simulink model "DC_motor_Real_sys_open"  (R2021b)
settings: Solver=FixedStepAuto  StartTime=0.0  StopTime=10.0  RelTol=1e-3
undefined symbols (not defined in the file): sigbuilder_block
libraries: arduinolib x2, arduinosensorlib x1
settings Model: ExtModeTrigDuration=2  Creator=Marco Milanesi  LastModifiedBy=Marco Milanesi
settings OptimizationCC: EnhancedBackFolding=on  PassReuseOutputArgsAs=Individual arguments  ZeroExternalMemoryAtStartup=off  ZeroInternalMemoryAtStartup=off  MaxStackSize=64  OptimizeBlockOrder=speed  DifferentSizesBufferReuse=on  OptimizationCustomize=off  EfficientTunableParamExpr=on
settings DebuggingCC: ParameterTunabilityLossMsg=error
settings HardwareCC: ProdBitPerInt=16  ProdBitPerPointer=16  ProdBitPerSizeT=16  ProdBitPerPtrDiffT=16  ProdLargestAtomicFloat=None  ProdWordSize=8  ProdHWDeviceType=Atmel->AVR  UseEmbeddedCoderFeatures=off  UseSimulinkCoderFeatures=off
settings SFSimCC: MATLABDynamicMemAlloc=off
settings RTWCC: Description=Embedded Coder  SystemTargetFile=ert.tlc  HardwareBoard=Arduino Uno  TemplateMakefile=ert_default_tmf  Toolchain=Arduino AVR
settings CodeAppCC: ForceParamTrailComments=on  IgnoreCustomStorageClasses=off  OperatorAnnotations=on  SimulinkDataObjDesc=on  SFDataObjDesc=on  InsertBlockDesc=on
settings ERTTargetCC: SupportContinuousTime=on  SupportNonInlinedSFcns=on  SupportVariableSizeSignals=on  ExtModeTransport=3  ExtModeStaticAlloc=on  ExtModeStaticAllocSize=250  ExtModeMexFile=ext_xcp  ExtModeIntrfLevel=Level2 - Open

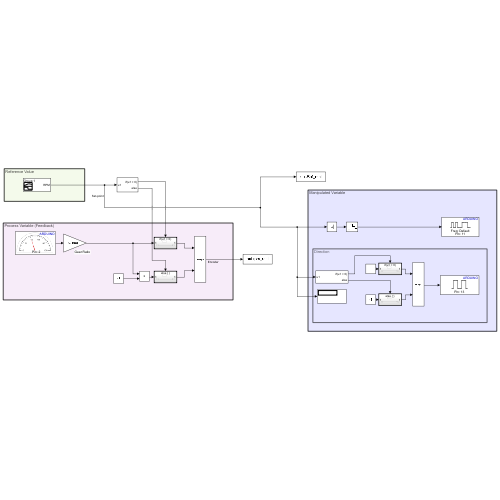
[thumbnail: Simulink's stored preview of the top-level diagram]
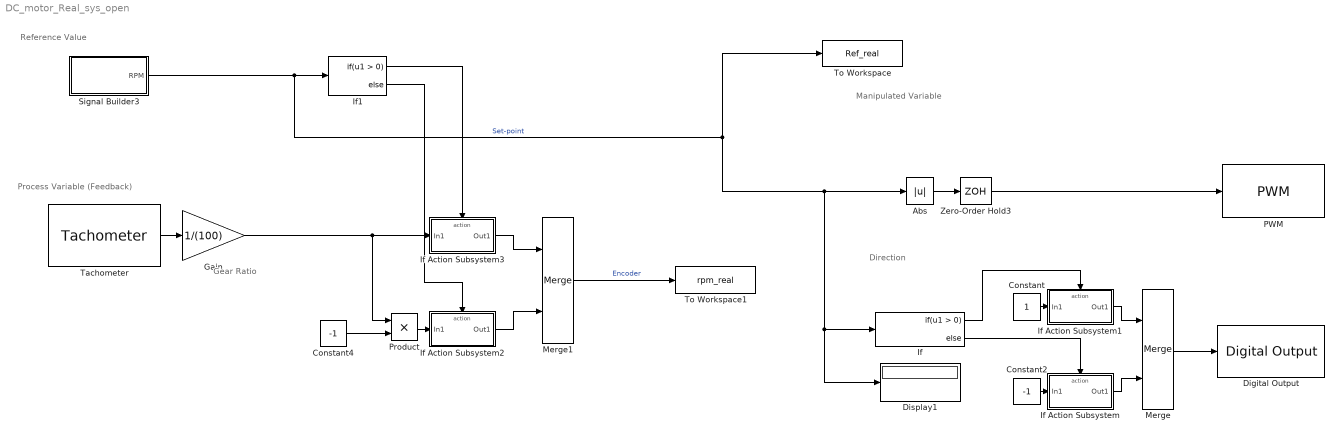
== system DC_motor_Real_sys_open ==
  note: Reference Value
  note: Process Variable (Feedback)
  note: Direction
  note: Manipulated Variable
  note: Gear Ratio
  Abs : Abs
  Constant : Constant
  Constant2 : Constant  Value=-1
  Constant4 : Constant  Value=-1
  Digital Output : arduinolib/Digital Output  pinNumber=13  Direction=output  blockPlatform=arduino
  Display1 : Display
  Gain : Gain  Gain=1/(100)  OutDataTypeStr=double
  If : If
  If Action Subsystem : Subsystem  TreatAsAtomicUnit=on
  If Action Subsystem1 : Subsystem  TreatAsAtomicUnit=on
  If Action Subsystem2 : Subsystem  TreatAsAtomicUnit=on
  If Action Subsystem3 : Subsystem  TreatAsAtomicUnit=on
  If1 : If
  Merge : Merge
  Merge1 : Merge
  PWM : arduinolib/PWM  pinNumber=11  frequencyType=Default  desiredFrequency=490.2  achievableFrequency=490.2
  Product : Product
  Signal Builder3 : Subsystem  Tag=STV Subsys  LoadFcn=sigbuilder_block('load');  StartFcn=sigbuilder_block('start');  StopFcn=sigbuilder_block('stop');  ClipboardFcn=sigbuilder_block('clipboard');  mask(Sigbuilder block){tuvar=[0:10]}
      mask help: Simulink:masks:SigbuilderBlock_MD
      mask init:
      | if ~strcmp(get_param(bdroot(gcbh),'SimulationStatus'),'stopped') tuvar = sigbuilder_block('maskInit'); end
      settings: CopyFcn=sigbuilder_block('copy');  DeleteFcn=sigbuilder_block('delete');  ModelCloseFcn=sigbuilder_block('modelClose');  PreSaveFcn=sigbuilder_block('preSave');  PauseFcn=sigbuilder_block('pause');  ContinueFcn=sigbuilder_block('continue');  NameChangeFcn=sigbuilder_block('namechange');  OpenFcn=sigbuilder_block('open',[43.4717 156.226 635.774 277.132 ]);  CloseFcn=sigbuilder_block('close');
      mask Display: plot(0, 0, 100, 100,[2, 2, 32, 32, 2], [68, 8, 8, 68, 68],[32, 2], [38, 38], [32, 19, 2],[53, 60, 44], [32, 17, 17, 2],[16, 16, 31, 31]);txt = getActiveGroup(gcbh);text(2, 100, txt,'verticalAlignment', 'top');
  Tachometer : arduinosensorlib/Tachometer  PinNumber=2  InterruptMode=RISING  PulseCountperRotation=1  SampleTime=0.1  blockPlatform=ARDUINO
      settings: SourceProductBaseCode=ARDUINO
  To Workspace : ToWorkspace  VariableName=Ref_real  SaveFormat=Structure With Time  SampleTime=-1
  To Workspace1 : ToWorkspace  VariableName=rpm_real  SaveFormat=Structure With Time  SampleTime=-1
  Zero-Order Hold3 : ZeroOrderHold  SampleTime=-1
  wires:
  If1/1 -> If Action Subsystem3/Action
  If Action Subsystem3/1(Out1) -> Merge1/1
  Signal Builder3/1(RPM) -> To Workspace/1, Abs/1, If/1, Display1/1, If1/1  "Set-point"
  If Action Subsystem/1(Out1) -> Merge/2
  If1/2 -> If Action Subsystem2/Action
  If Action Subsystem2/1(Out1) -> Merge1/2
  Product/1 -> If Action Subsystem2/1(In1)
  Merge1/1 -> To Workspace1/1  "Encoder"
  Constant4/1 -> Product/2
  Gain/1 -> Product/1, If Action Subsystem3/1(In1)
  If Action Subsystem1/1(Out1) -> Merge/1
  Zero-Order Hold3/1 -> PWM/1
  If/2 -> If Action Subsystem/Action
  Tachometer/1 -> Gain/1
  Constant2/1 -> If Action Subsystem/1(In1)
  Constant/1 -> If Action Subsystem1/1(In1)
  Merge/1 -> Digital Output/1
  If/1 -> If Action Subsystem1/Action
  Abs/1 -> Zero-Order Hold3/1

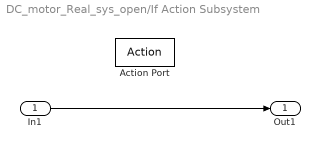
== system DC_motor_Real_sys_open/If Action Subsystem ==
  In1 : Inport
  Action Port : ActionPort  ActionPortLabel=else
  Out1 : Outport
  wires:
  In1/1 -> Out1/1

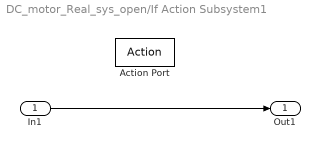
== system DC_motor_Real_sys_open/If Action Subsystem1 ==
  In1 : Inport
  Action Port : ActionPort  ActionPortLabel=if(u1 > 0)
  Out1 : Outport
  wires:
  In1/1 -> Out1/1

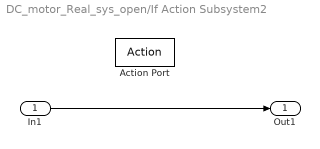
== system DC_motor_Real_sys_open/If Action Subsystem2 ==
  In1 : Inport
  Action Port : ActionPort  ActionPortLabel=else
  Out1 : Outport
  wires:
  In1/1 -> Out1/1

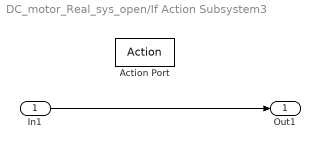
== system DC_motor_Real_sys_open/If Action Subsystem3 ==
  In1 : Inport
  Action Port : ActionPort  ActionPortLabel=if(u1 > 0)
  Out1 : Outport
  wires:
  In1/1 -> Out1/1

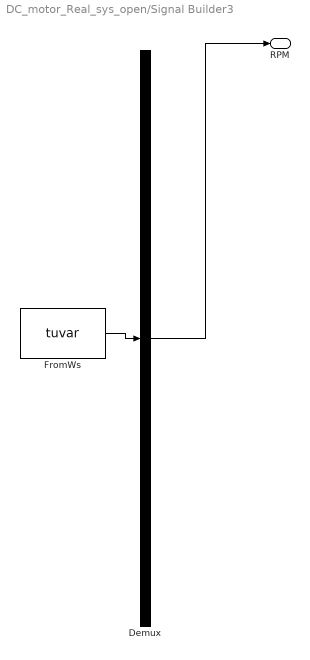
== system DC_motor_Real_sys_open/Signal Builder3 ==
  Demux : Demux  Tag=STV Demux  Outputs=1
      settings: DisplayOption=none
  FromWs : FromWorkspace  Tag=STV FromWs  VariableName=tuvar
      SigBuilderData=|
      | common.afterFinalStr = 'Extrapolate'
      | common.sampleTime = 0
      | dataSet.timeRange = [0 100]
      | dataSet.name = 'Group 1'
      | sbobj.Groups.Name = 'Group 1'
      | sbobj.Groups.Signals.Name = 'RPM'
      | sbobj.Groups.Signals.XData = [0 5 5 10 10 15 15 20 20 25 25 30 30 35 35 39.95 40 45 45 50 50 55 55 60 60 65 65 70 70 75 75 80 80 85 85 95 95 100]
      | sbobj.Groups.Signals.YData = [0 0 100 100 -300 -300 -150 -150 400 400 200 200 -500 -500 -350 -350 330 330 -100 -100 -250 -250 -200 -200 500 500 100 100 335 335 200 200 -340 -340 -150 -150 100 100]
      | sbobj.Groups.TimeRange = [0 100]
  RPM : Outport  Tag=STV Outport
  wires:
  Demux/1 -> RPM/1
  FromWs/1 -> Demux/1
